simulink model "atc_ut"  (Simulink 8.1)
settings: Solver=FixedStepDiscrete  StartTime=0.0  StopTime=Inf  FixedStep=0.005  RelTol=1e-3
PostLoadFcn:
  | , if any(exist('dsrtsu_mdlpostloadfcn', 'file') == [2, 3, 6]), try dsrtsu_mdlpostloadfcn('Execute', bdroot); catch fprintf('Error in PostLoadFcn (dsrtsu_mdlpostloadfcn) for model "%s":\n %s\n', bdroot, lasterr); end, end,
libraries: siltestlib x7, atc x1
settings Model: DSRTSU_INTERNAL_RTI_VER=450  DSRTSU_INTERNAL_RTI_TYPE=rti1401  RTICANMMDATA=struct('GeneralSetupData',struct('modelroot','D:\ELN150201_TAIWAN\trunk\AdasDragon\software\sw_development\arch\app\jud','generalsettings',struct('filesettings',struct('destfolder',struct('Name','RTICANMM_FILES','Check',1),'buildfolder',struct('Name','.','Check',1),'AbsDestfolder',struct('Name','D:\ELN150201_TAIWAN\trunk\AdasDragon\software\sw_development\arch\app\jud\RTICANMM_FILES'),'AbsBuildfolder',struct('Name','D:\ELN150201_TAIWAN\trunk\AdasDragon\software\sw_development\arch\app\jud'))),'options',struct('addpaths',1,'rmpaths',1,'addtrcexclusion',logical(1),'cannavigator',struct('checkmonitoring',0),'show_usrtrc',0,'use_usrtrc',0),'advanced',struct('options',[1 1 1 1 1 1 1 1 1 1 1 1 1 1 1 1 1 1 1 1 1 1 1 1 1 1 1 1 1 1 1 1 1 1 1 1 1 1 1 1 1 1 1 1 1 1 1 1 1 1 1 1 1 1 1 1 1 1 1 1 1 1 1 1 1 1 1 1 1 1 1 1 1 1 1 1 1 1 1 1 1 1 1 1 1 1 1 1 1 1 1 1 1 1 1 1 1 1 1 1]),'MPSetup',{{}},'modelname','atc_ut','block','atc_ut'))  DSRTSU_INTERNAL_RTIFPGA=40  Creator=AT015411  LastModifiedBy=AT015555  BufferReuse=off
settings DataIOCC: SignalLoggingSaveFormat=Dataset
settings OptimizationCC: BlockReduction=off  OptimizeBlockIOStorage=off  BufferReuse=off  ExpressionFolding=off  ExpressionDepthLimit=128  LocalBlockOutputs=off
settings DebuggingCC: FcnCallInpInsideContextMsg=EnableAllAsError
settings HardwareCC: ProdIntDivRoundTo=Zero  ProdEndianess=BigEndian  ProdHWDeviceType=Generic->Custom  TargetIntDivRoundTo=Zero  TargetEndianess=BigEndian  TargetHWDeviceType=Generic->Custom
settings RTWCC: SystemTargetFile=rti1005.tlc  MakeCommand=make_rti  TemplateMakefile=rti1005.tmf  Description=dSPACE DS1005 Hardware Platform  ProcessScript=rti1005_make_rtw_hook
settings STFCustomTargetCC: CodeReplacementLibrary=ANSI_C  ParMdlRefBuildCompliant=on  GeneratePreprocessorConditionals=Disable all  MatFileLogging=on  SystemTargetFile=rti1005.tlc
settings GRTTargetCC: CompOptLevelCompliant=off  ConcurrentExecutionCompliant=off  ExtModeMexFile=noextcomm
settings CustomProperty: DataType=RTWOptions_EnumType_C__Program Files (x86)_dSPACE RCPHIL 2014-B_MATLAB_RTI_RTI1401_TLC_rti1005_1InitialSimState  Value=RUN
settings EnumStrPairs: String=RUN

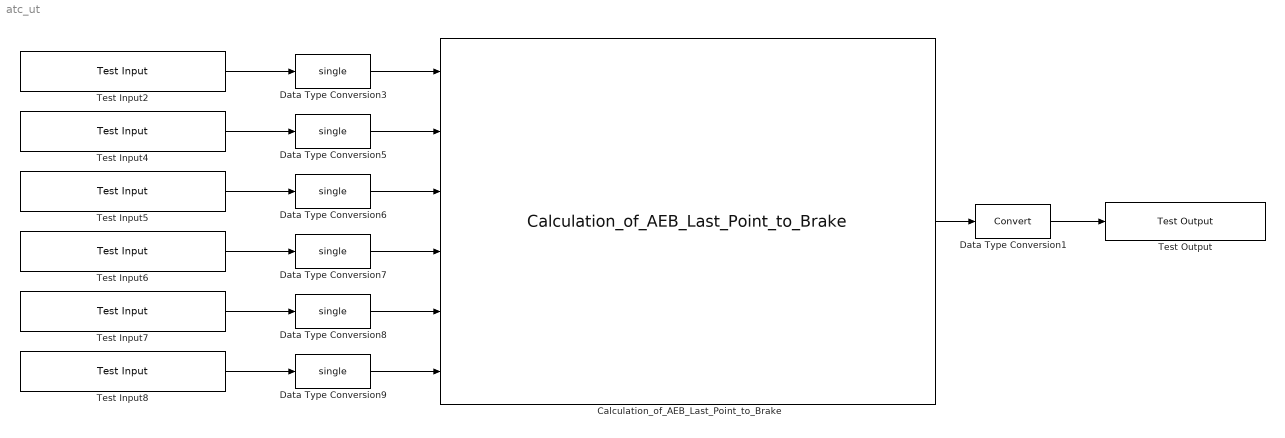
== system atc_ut ==
  Calculation_of_AEB_Last_Point_to_Brake : atc/Calculation_of_AEB_Last_Point_to_Brake
  Data Type Conversion1 : DataTypeConversion
  Data Type Conversion{3,5..9} (6 alike) : DataTypeConversion  OutDataTypeStr=single
  Test Input2 : siltestlib/Test Input  varname=VJUD_FreeRunningTime_sec  sampletime=0.005
  Test Input4 : siltestlib/Test Input  varname=VIFO_AEBTargetVehRelSpeedX_mps  sampletime=0.005
  Test Input5 : siltestlib/Test Input  varname=VDINR_VehSpd_mps  sampletime=0.005
  Test Input6 : siltestlib/Test Input  varname=VJUD_AEBMCVehAbsSpdX_mps  sampletime=0.005
  Test Input7 : siltestlib/Test Input  varname=VJUD_AEBMCLongAcc_mps2  sampletime=0.005
  Test Input8 : siltestlib/Test Input  varname=VIFO_AEBTGap_s  sampletime=0.005
  Test Output : siltestlib/Test Output  varname=VJUD_PointToBrake_m  sampletime=-1
  wires:
  Data Type Conversion1/1 -> Test Output/1
  Calculation_of_AEB_Last_Point_to_Brake/1 -> Data Type Conversion1/1
  Test Input2/1 -> Data Type Conversion3/1
  Data Type Conversion3/1 -> Calculation_of_AEB_Last_Point_to_Brake/1
  Test Input4/1 -> Data Type Conversion5/1
  Data Type Conversion5/1 -> Calculation_of_AEB_Last_Point_to_Brake/2
  Test Input5/1 -> Data Type Conversion6/1
  Data Type Conversion6/1 -> Calculation_of_AEB_Last_Point_to_Brake/3
  Test Input6/1 -> Data Type Conversion7/1
  Data Type Conversion7/1 -> Calculation_of_AEB_Last_Point_to_Brake/4
  Test Input7/1 -> Data Type Conversion8/1
  Data Type Conversion8/1 -> Calculation_of_AEB_Last_Point_to_Brake/5
  Test Input8/1 -> Data Type Conversion9/1
  Data Type Conversion9/1 -> Calculation_of_AEB_Last_Point_to_Brake/6
